simulink model "xu_sim_2019"  (R2019a)
settings: Solver=ode23s  StartTime=0.0  StopTime=tsim  RelTol=1e-2
values from neighbouring files (symbols this model uses):
  A_1_low = 0.50    (= 0.5)    [main_simulation.m]    (also in main_xu_simulink.m)
  A_1_mid = A_1_max - A_1_min    (= 0.79)    [main_simulation.m]    (also in main_xu_simulink.m)
  A_1_min = 0.21    [main_simulation.m]    (also in main_xu_simulink.m)
  A_1_upp = 1    [main_simulation.m]    (also in main_xu_simulink.m)
  Estrategia = 1    [main_simulation.m]    (also in main_xu_simulink.m)
  G_1_low = 0.30    (= 0.3)    [main_simulation.m]    (also in main_xu_simulink.m)
  G_1_mid = G_1_max - G_1_min    (= 0.4)    [main_simulation.m]    (also in main_xu_simulink.m)
  G_1_min = 0.2    [main_simulation.m]    (also in main_xu_simulink.m)
  G_1_upp = 0.50    (= 0.5)    [main_simulation.m]    (also in main_xu_simulink.m)
  mu_set = 0.13    [avoidCurveFit.m]    (also in funObj.m; main.m = 0.29; main_ajuste.m; main_simulation.m = 0.31)
  N_1_low = 0    [main_simulation.m]    (also in main_xu_simulink.m)
  N_1_max = 300    [main_simulation.m]    (also in main_xu_simulink.m)
  N_1_min = 300    [main_simulation.m]    (also in main_xu_simulink.m)
  N_1_upp = 0.30    (= 0.3)    [main_simulation.m]    (also in main_xu_simulink.m)
  PI_Kd = 0    [main_simulation.m]    (also in main_xu_simulink.m)
  PI_Kd_2 = 0    [main_simulation.m]    (also in main_xu_simulink.m)
  PI_Ki = 1163.22932064265    (= 1163.22932064)    [main_simulation.m]    (also in main_xu_simulink.m)
  PI_Ki_2 = 0.06    [main_simulation.m]    (also in main_xu_simulink.m)
  PI_Kp = 1.87082881181595    (= 1.87082881182)    [main_simulation.m]    (also in main_xu_simulink.m)
  PI_Kp_2 = 13.0    (= 13)    [main_simulation.m]    (also in main_xu_simulink.m)
  Sfeed = 550    [avoidCurveFit.m]    (also in funObj.m; main.m; main_ajuste.m; main_simulation.m)
  spO2 = 0.3*O2s    (= 0.00238555038055)    [main_simulation.m]    (also in main_xu_simulink.m = 0.3*O2s)
  Ts = 1/60    (= 0.0166666666667)    [main_simulation.m]    (also in main_xu_simulink.m)
  u_1_low = 0    [main_simulation.m]    (also in main_xu_simulink.m)
  u_1_upp = 1    [main_simulation.m]    (also in main_xu_simulink.m)
  Vin = 0.3    [avoidCurveFit.m]    (also in funObj.m; main.m = 6.8; main_ajuste.m; main_simulation.m = 6.8)
  Xin = 5    [avoidCurveFit.m]    (also in funObj.m; main.m = 0.4; main_ajuste.m; main_simulation.m = 0.4)
  YS_ox_X = 0.51    [main.m]    (also in main_ajuste.m; main_simulation.m; xu_model.m = k(1); xu_parameters.m)
undefined symbols (not defined in the file or in its folder): magnitude
libraries: simulink x6
settings Model: Creator=dnavalos  LastModifiedBy=dnavalos
settings DebuggingCC: SFMachineParentedDataDiag=error

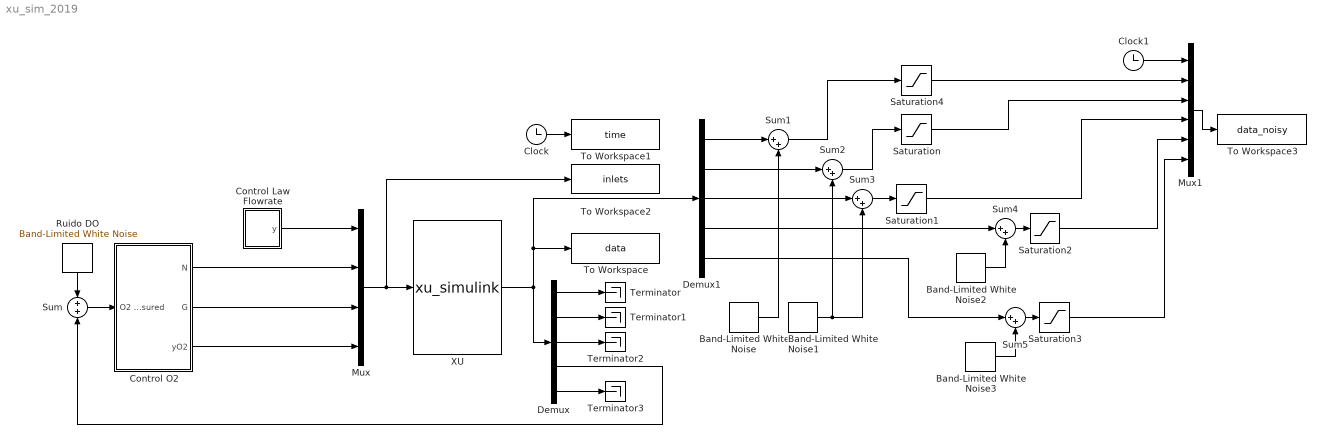
== system xu_sim_2019 ==
  Band-Limited White Noise : simulink/Sources/Band-Limited White Noise  Cov=[10]  Ts=0.2  seed=[23341]
  Band-Limited White Noise1 : simulink/Sources/Band-Limited White Noise  Cov=[1e-4]  Ts=0.2  seed=[23341]
  Band-Limited White Noise2 : simulink/Sources/Band-Limited White Noise  Cov=[1e-8]  Ts=0.2  seed=[23341]
  Band-Limited White Noise3 : simulink/Sources/Band-Limited White Noise  Cov=[0.01]  Ts=0.2  seed=[23341]
  Clock : Clock
  Clock1 : Clock
  Control Law Flowrate : Subsystem
  Control O2 : Subsystem
  Demux : Demux  Outputs=5
  Demux1 : Demux  Outputs=5
  Mux : Mux
  Mux1 : Mux  Inputs=6
  Ruido DO : simulink/Sources/Band-Limited White Noise  Cov=sigma_DO  Ts=Ts  seed=[23341]
  Saturation{,1..4} (5 alike) : Saturate  UpperLimit=inf  LowerLimit=0
  Sum : Sum
  Sum{1..5} (5 alike) : Sum  Inputs=|++
  Terminator{,1..3} (4 alike) : Terminator
  To Workspace : ToWorkspace  VariableName=data  SampleTime=-1
  To Workspace1 : ToWorkspace  VariableName=time  SampleTime=-1
  To Workspace2 : ToWorkspace  VariableName=inlets  SampleTime=-1
  To Workspace3 : ToWorkspace  VariableName=data_noisy  SampleTime=1
  XU : S-Function  FunctionName=xu_simulink  SFunctionDeploymentMode=off  EnableBusSupport=off
      mask Display: image('reactor.jpg'); % Use "Edit Image" on toolstrip to change.
  wires:
  XU/1 -> Demux1/1, To Workspace/1, Demux/1
  Clock/1 -> To Workspace1/1
  Control Law Flowrate/1(y) -> Mux/1
  Mux/1 -> To Workspace2/1, XU/1
  Control O2/1(N) -> Mux/2
  Control O2/2(G) -> Mux/3
  Control O2/3(yO2) -> Mux/4
  Demux/4 -> Sum/2
  Sum/1 -> Control O2/1(O2 measured)
  Ruido DO/1 -> Sum/1
  Demux/5 -> Terminator3/1
  Demux/3 -> Terminator2/1
  Demux/2 -> Terminator1/1
  Demux/1 -> Terminator/1
  Demux1/1 -> Sum1/1
  Demux1/2 -> Sum2/1
  Band-Limited White Noise/1 -> Sum1/2
  Sum1/1 -> Saturation4/1
  Demux1/3 -> Sum3/1
  Demux1/5 -> Sum5/1
  Demux1/4 -> Sum4/1
  Sum2/1 -> Saturation/1
  Band-Limited White Noise1/1 -> Sum3/2, Sum2/2
  Saturation/1 -> Mux1/3
  Sum3/1 -> Saturation1/1
  Saturation1/1 -> Mux1/4
  Saturation2/1 -> Mux1/5
  Sum4/1 -> Saturation2/1
  Band-Limited White Noise2/1 -> Sum4/2
  Sum5/1 -> Saturation3/1
  Band-Limited White Noise3/1 -> Sum5/2
  Saturation3/1 -> Mux1/6
  Saturation4/1 -> Mux1/2
  Mux1/1 -> To Workspace3/1
  Clock1/1 -> Mux1/1

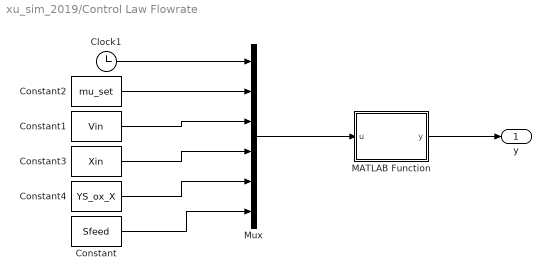
== system xu_sim_2019/Control Law Flowrate ==
  Clock1 : Clock
  Constant : Constant  Value=Sfeed
  Constant1 : Constant  Value=Vin
  Constant2 : Constant  Value=mu_set
  Constant3 : Constant  Value=Xin
  Constant4 : Constant  Value=YS_ox_X
  MATLAB Function : MATLAB Function  TreatAsAtomicUnit=on
  Mux : Mux  Inputs=6
  y : Outport
  wires:
  Constant/1 -> Mux/6
  Constant3/1 -> Mux/4
  Clock1/1 -> Mux/1
  Constant2/1 -> Mux/2
  Constant1/1 -> Mux/3
  Constant4/1 -> Mux/5
  Mux/1 -> MATLAB Function/1(u)
  MATLAB Function/1(y) -> y/1

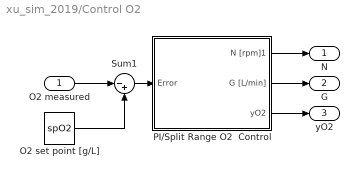
== system xu_sim_2019/Control O2 ==
  O2 measured : Inport
  O2 set point [g/L] : Constant  Value=spO2
  PI/Split Range O2  Control : Subsystem
  Sum1 : Sum  Inputs=|-+
  N : Outport  VectorParamsAs1DForOutWhenUnconnected=off
  G : Outport  Port=2  VectorParamsAs1DForOutWhenUnconnected=off
  yO2 : Outport  Port=3  VectorParamsAs1DForOutWhenUnconnected=off
  wires:
  PI/Split Range O2  Control/1(N [rpm]1) -> N/1
  PI/Split Range O2  Control/2(G [L/min]) -> G/1
  O2 measured/1 -> Sum1/1
  O2 set point [g/L]/1 -> Sum1/2
  PI/Split Range O2  Control/3("yO2 ") -> yO2/1
  Sum1/1 -> PI/Split Range O2  Control/1(Error)

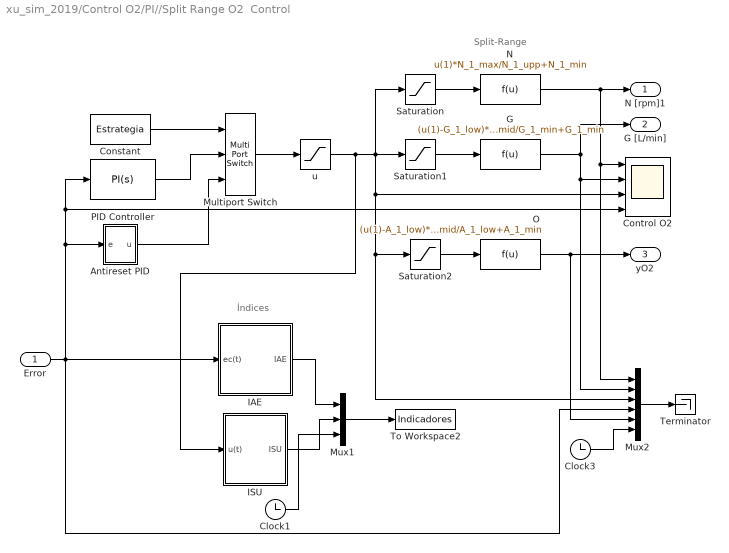
== system xu_sim_2019/Control O2/PI//Split Range O2  Control ==
  note: Índices
  note: Split-Range
  Error : Inport
  Antireset PID : Subsystem  mask(Antireset PID){G=PI_Kp_2, ti=PI_Ki_2, td=PI_Kd_2, a=0.5, U=1, L=0}
      mask prompts: G "Controller Gain"; ti "Integral Time Constant"; td "Derivative Time Constant"; a "Alpha"; U "Saturation Upper Limit"; L "Saturation Lower Limit"
      mask help: Enter expression for Controller Gain, Integral Time Constant, Derivative Time Constant, Alpha Constant, Saturation Upper Constant, and Saturation Lower Constant terms.
  Clock1 : Clock
  Clock3 : Clock
  Constant : Constant  Value=Estrategia
  Control O2 : Scope  NumInputPorts=4
  G : Fcn  Expr=(u(1)-G_1_low)*G_1_mid/G_1_min+G_1_min
  IAE : Subsystem
  ISU : Subsystem
  Multiport Switch : MultiPortSwitch  Inputs=2
  Mux1 : Mux  Inputs=3
  Mux2 : Mux  Inputs=6
  N : Fcn  Expr=u(1)*N_1_max/N_1_upp+N_1_min
  O : Fcn  Expr=(u(1)-A_1_low)*A_1_mid/A_1_low+A_1_min
  PID Controller : simulink/Continuous/PID Controller  Controller=PI  Form=Parallel  TimeDomain=Continuous-time  SampleTime=-1  IntegratorMethod=Forward Euler  FilterMethod=Forward Euler  ControllerParametersSource=internal  P=PI_Kp  I=PI_Ki  D=PI_Kd  UseFilter=on  N=479.898765366224  TunerSelectOption=Transfer Function Based (PID Tuner App)  InitialConditionSource=internal  InitialConditionForIntegrator=-48.255  InitialConditionForFilter=0  DifferentiatorICPrevScaledInput=0  ExternalReset=none  TrackingMode=off  Kt=1  LimitOutput=on  UpperSaturationLimit=1  LowerSaturationLimit=0  LinearizeAsGain=off  AntiWindupMode=back-calculation  Kb=1  POutMin=[]  POutMax=[]  IOutMin=[]  IOutMax=[]  DOutMin=[]  DOutMax=[]  NOutMin=[]  NOutMax=[]  SumOutMin=[]  SumOutMax=[]  SaturationOutMin=[]  SaturationOutMax=[]  PParamMin=[]  PParamMax=[]  IParamMin=[]  IParamMax=[]  DParamMin=[]  DParamMax=[]  NParamMin=[]  NParamMax=[]  KbParamMin=[]  KbParamMax=[]  KtParamMin=[]  KtParamMax=[]  KbOutMin=[]  KbOutMax=[]  KtOutMin=[]  KtOutMax=[]  IntegratorOutMin=[]  IntegratorOutMax=[]  FilterOutMin=[]  FilterOutMax=[]  SumI1OutMin=[]  SumI1OutMax=[]  SumI2OutMin=[]  SumI2OutMax=[]  SumI3OutMin=[]  SumI3OutMax=[]  SumI4OutMin=[]  SumI4OutMax=[]  SumDOutMin=[]  SumDOutMax=[]  DifferentiatorOutMin=[]  DifferentiatorOutMax=[]  FilterDiffOutCoefMin=[]  FilterDiffOutCoefMax=[]  ReciprocalOutMin=[]  ReciprocalOutMax=[]  SumDenOutMin=[]  SumDenOutMax=[]  SumNumOutMin=[]  SumNumOutMax=[]  DivideOutMin=[]  DivideOutMax=[]  IntegratorContinuousStateAttributes=''  IntegratorStateMustResolveToSignalObject=off  IntegratorRTWStateStorageClass=Auto  FilterContinuousStateAttributes=''  FilterStateMustResolveToSignalObject=off  FilterRTWStateStorageClass=Auto  ParallelPVariant=InternalParameters  IdealPVariant=Disabled  IVariant=InternalParameters  DVariant=Disabled  IntegratorVariant=Continuous  SatVariant=Enabled  AWVariant=BackCalculation  PCopyVariant=Disabled  TRVariant=Disabled  FdbkBlocksVariant=Forward  IdealPFdbkVariant=Disabled  SatFdbkVariant=Disabled  DerivativeFilterVariant=Disabled  NVariant=Disabled  NCopyVariant=Disabled_SignalSpec  FilterICVariant=Disabled  IntegratorICVariant=InternalICs  ExternalResetVariant=Disabled  TRSumVariant=Passthrough  SumFdbkVariant=Disabled  SumVariant=Sum_PI
  Saturation : Saturate  UpperLimit=N_1_upp  LowerLimit=N_1_low
  Saturation1 : Saturate  UpperLimit=G_1_upp  LowerLimit=G_1_low
  Saturation2 : Saturate  UpperLimit=A_1_upp  LowerLimit=A_1_low
  Terminator : Terminator
  To Workspace2 : ToWorkspace  VariableName=Indicadores  SampleTime=-1
  u : Saturate  UpperLimit=u_1_upp  LowerLimit=u_1_low
  N [rpm]1 : Outport  VectorParamsAs1DForOutWhenUnconnected=off
  G [L/min] : Outport  Port=2  VectorParamsAs1DForOutWhenUnconnected=off
  "yO2 " : Outport  Port=3  VectorParamsAs1DForOutWhenUnconnected=off
  wires:
  Saturation2/1 -> O/1
  Constant/1 -> Multiport Switch/1
  Clock3/1 -> Mux2/6
  N/1 -> N [rpm]1/1, Mux2/1, Control O2/1
  Multiport Switch/1 -> u/1
  ISU/1(ISU) -> Mux1/2
  IAE/1(IAE) -> Mux1/1
  Clock1/1 -> Mux1/3
  Mux1/1 -> To Workspace2/1
  Mux2/1 -> Terminator/1
  PID Controller/1 -> Multiport Switch/2
  Saturation1/1 -> G/1
  Saturation/1 -> N/1
  O/1 -> Mux2/5, "yO2 "/1
  Antireset PID/1(u) -> Multiport Switch/3
  u/1 -> ISU/1(u(t)), Saturation/1, Saturation1/1, Mux2/3, Saturation2/1, Control O2/3
  G/1 -> G [L/min]/1, Mux2/2, Control O2/2
  Error/1 -> PID Controller/1, Control O2/4, Antireset PID/1(e), Mux2/4, IAE/1(ec(t))

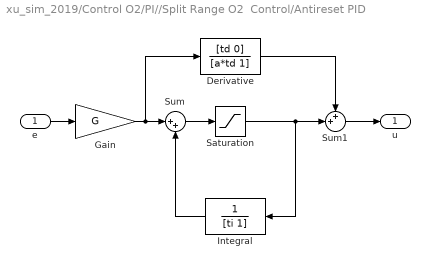
== system xu_sim_2019/Control O2/PI//Split Range O2  Control/Antireset PID ==
  e : Inport
  Derivative : TransferFcn  Numerator=[td 0]  Denominator=[a*td 1]
  Gain : Gain  Gain=G  SaturateOnIntegerOverflow=on  OutDataTypeStr=Inherit: Same as input  ParamDataTypeStr=Inherit: Same as input
  Integral : TransferFcn  Denominator=[ti 1]
  Saturation : Saturate  UpperLimit=U  LowerLimit=L
  Sum : Sum  Inputs=|++  InputSameDT=on  SaturateOnIntegerOverflow=on  OutDataTypeStr=Inherit: Same as first input
  Sum1 : Sum  Inputs=++|  InputSameDT=on  SaturateOnIntegerOverflow=on  OutDataTypeStr=Inherit: Same as first input
  u : Outport  VectorParamsAs1DForOutWhenUnconnected=off
  wires:
  Derivative/1 -> Sum1/1
  Sum1/1 -> u/1
  Saturation/1 -> Integral/1, Sum1/2
  e/1 -> Gain/1
  Integral/1 -> Sum/2
  Sum/1 -> Saturation/1
  Gain/1 -> Derivative/1, Sum/1

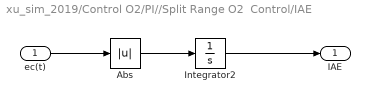
== system xu_sim_2019/Control O2/PI//Split Range O2  Control/IAE ==
  ec(t) : Inport
  Abs : Abs
  Integrator2 : Integrator
  IAE : Outport  VectorParamsAs1DForOutWhenUnconnected=off
  wires:
  Abs/1 -> Integrator2/1
  ec(t)/1 -> Abs/1
  Integrator2/1 -> IAE/1

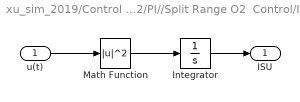
== system xu_sim_2019/Control O2/PI//Split Range O2  Control/ISU ==
  u(t) : Inport
  Integrator : Integrator
  Math Function : Math  Operator=magnitude^2  SaturateOnIntegerOverflow=on
  ISU : Outport  VectorParamsAs1DForOutWhenUnconnected=off
  wires:
  Integrator/1 -> ISU/1
  u(t)/1 -> Math Function/1
  Math Function/1 -> Integrator/1

== matlab function xu_sim_2019/Control Law Flowrate/MATLAB Function ==
  data: u input; y output
function y = fcn(u)
mu_set = u(2); Vin = u(3); Xin = u(4); YS_ox_X = u(5); Sfeed = u(6);
t = u(1);

y = mu_set*Vin*Xin*exp(mu_set*t)/(YS_ox_X*Sfeed);
end
